simulink model "teste_modelo"  (R2017a)
settings: Solver=VariableStepAuto  StartTime=0.0  StopTime=300  RelTol=1e-3
values from neighbouring files (symbols this model uses):
  den = [den,-theta(i)]    [MQARX.m]
  num = [num,0]    [MQARX.m]
undefined symbols (not defined in the file or in its folder): A2, A3, B2, B3, C2, C3, D2, D3, G10
settings Model: Creator=mateu  LastModifiedBy=mateu

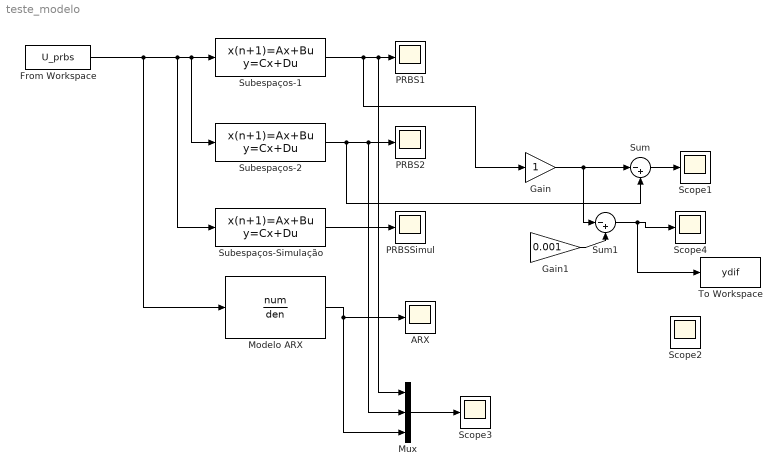
== system teste_modelo ==
  ARX : Scope
  From Workspace : FromWorkspace  VariableName=U_prbs  SampleTime=0.1
  Gain : Gain
  Gain1 : Gain  Gain=0.001
  Modelo ARX : TransferFcn  Numerator=num  Denominator=den
  Mux : Mux  Inputs=3
  PRBS1 : Scope
  PRBS2 : Scope
  PRBSSimul : Scope
  Scope{1..4} (4 alike) : Scope
  Subespaços-1 : DiscreteStateSpace  A=A2  B=B2  C=C2  D=D2  SampleTime=0.1
  Subespaços-2 : DiscreteStateSpace  A=A3  B=B3  C=C3  D=D3  SampleTime=0.1
  Subespaços-Simulação : DiscreteStateSpace  A=G10.A  B=G10.B  C=G10.C  D=G10.D  SampleTime=0.1
  Sum : Sum  Inputs=|-+
  Sum1 : Sum  Inputs=|-+
  To Workspace : ToWorkspace  VariableName=ydif  SampleTime=0.1
      settings: Save2DSignal=2-D array (concatenate along first dimension)
  wires:
  Subespaços-1/1 -> Gain/1, Mux/1, PRBS1/1
  Subespaços-2/1 -> Sum/2, Mux/2, PRBS2/1
  From Workspace/1 -> Modelo ARX/1, Subespaços-Simulação/1, Subespaços-2/1, Subespaços-1/1
  Subespaços-Simulação/1 -> PRBSSimul/1
  Mux/1 -> Scope3/1
  Modelo ARX/1 -> Mux/3, ARX/1
  ? -> Scope2/1, Gain1/1
  Sum/1 -> Scope1/1
  Gain/1 -> Sum1/1, Sum/1
  Gain1/1 -> Sum1/2
  Sum1/1 -> To Workspace/1, Scope4/1
